simulink model "zn_open"  (R2023b)
settings: Solver=VariableStepAuto  StartTime=0.0  StopTime=5  RelTol=1e-8
values from neighbouring files (symbols this model uses):
  D_hiv_fart = [M(3),rho_vann*Cd*A_z*Z_2]    [Alternative_Parameter.m]
settings Model: Creator=Anne Brit  LastModifiedBy=anneb

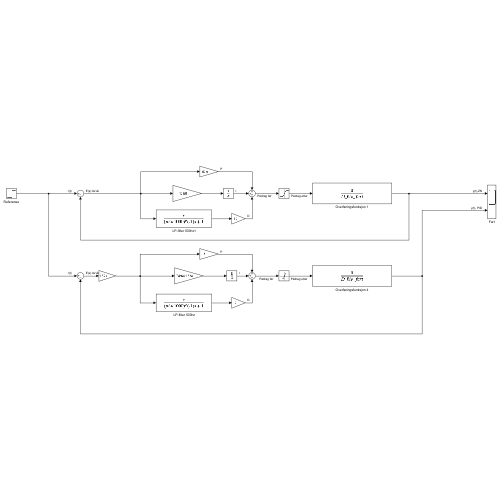
[thumbnail: Simulink's stored preview of the top-level diagram]
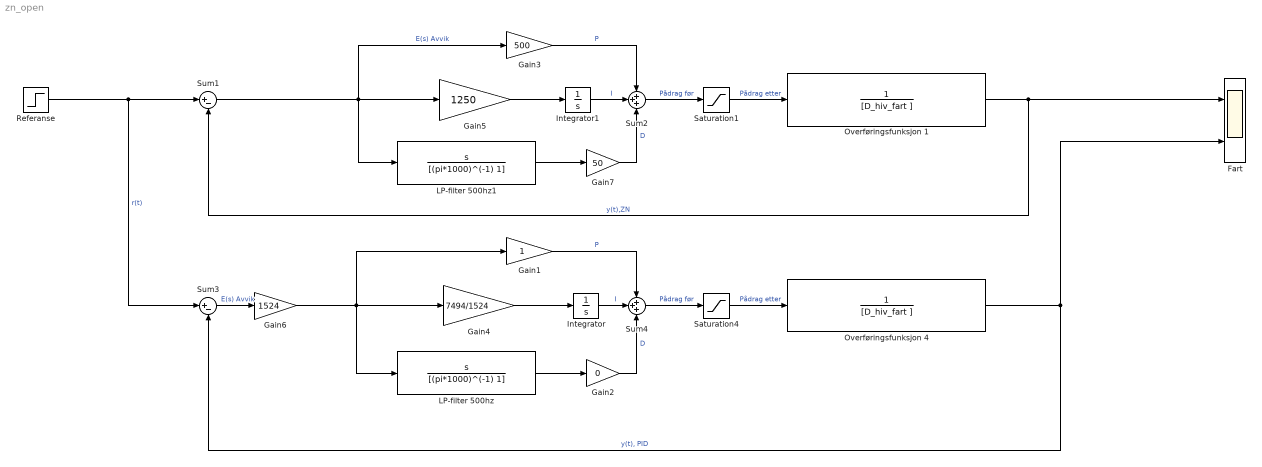
== system zn_open ==
  " LP-filter 500hz" : TransferFcn  Numerator=[1 0]  Denominator=[(pi*1000)^(-1) 1]
  " LP-filter 500hz1" : TransferFcn  Numerator=[1 0]  Denominator=[(pi*1000)^(-1) 1]
  Fart : Scope  NumInputPorts=2
  Gain1 : Gain
  Gain2 : Gain  Gain=0
  Gain3 : Gain  Gain=500
  Gain4 : Gain  Gain=7494/1524
  Gain5 : Gain  Gain=1250
  Gain6 : Gain  Gain=1524
  Gain7 : Gain  Gain=50
  Integrator : Integrator
  Integrator1 : Integrator
  Overføringsfunksjon 1 : TransferFcn  Denominator=[D_hiv_fart ]
  Overføringsfunksjon 4 : TransferFcn  Denominator=[D_hiv_fart ]
  Referanse : Step  After=0.0325  SampleTime=0
  Saturation1 : Saturate  UpperLimit=115  LowerLimit=-145
  Saturation4 : Saturate  UpperLimit=115  LowerLimit=-145
  Sum1 : Sum  Inputs=|+-
  Sum2 : Sum  Inputs=+++
  Sum3 : Sum  Inputs=|+-
  Sum4 : Sum  Inputs=+++
  wires:
  Sum4/1 -> Saturation4/1  "Pådrag før"
  Saturation4/1 -> Overføringsfunksjon 4/1  "Pådrag etter"
  Gain4/1 -> Integrator/1
  Overføringsfunksjon 4/1 -> Fart/2, Sum3/2  "y(t), PID"
  Gain1/1 -> Sum4/1  "P"
  Gain6/1 -> Gain1/1, Gain4/1, " LP-filter 500hz"/1
  Integrator/1 -> Sum4/2  "I"
  Sum3/1 -> Gain6/1  "E(s) Avvik"
  Gain2/1 -> Sum4/3  "D"
  " LP-filter 500hz"/1 -> Gain2/1
  Gain5/1 -> Integrator1/1
  Overføringsfunksjon 1/1 -> Sum1/2, Fart/1  "y(t),ZN"
  Gain3/1 -> Sum2/1  "P"
  Integrator1/1 -> Sum2/2  "I"
  Sum1/1 -> " LP-filter 500hz1"/1, Gain3/1, Gain5/1  "E(s) Avvik"
  Gain7/1 -> Sum2/3  "D"
  " LP-filter 500hz1"/1 -> Gain7/1
  Saturation1/1 -> Overføringsfunksjon 1/1  "Pådrag etter"
  Sum2/1 -> Saturation1/1  "Pådrag før"
  Referanse/1 -> Sum1/1, Sum3/1  "r(t)"
